simulink model "Group7_rotate"  (R2022a)
settings: Solver=FixedStepDiscrete  StartTime=0.0  StopTime=10  FixedStep=0.01  RelTol=1e-3
values from neighbouring files (symbols this model uses):
  axleLength = 0.136    [robotParameters.m]
  ticksPerRot = 20    [robotParameters.m]
  wheelR = 0.031    [robotParameters.m]
undefined symbols (not defined in the file or in its folder): DiscIntNeverNeededParam, InputPWM, lineLength, WheelSpeed
libraries: mobileRoboticsTrainingLib x4, slpidlib x1
settings Model: Creator=heath  LastModifiedBy=heath

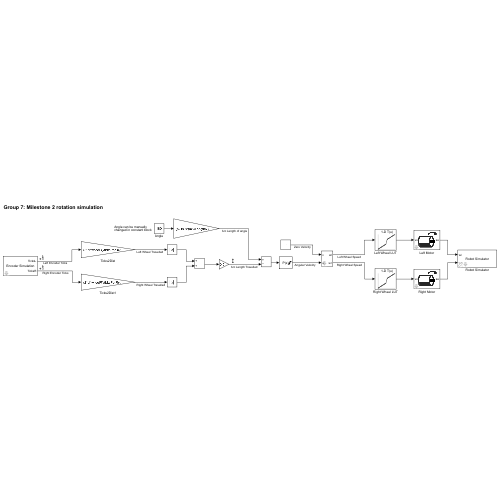
[thumbnail: Simulink's stored preview of the top-level diagram]
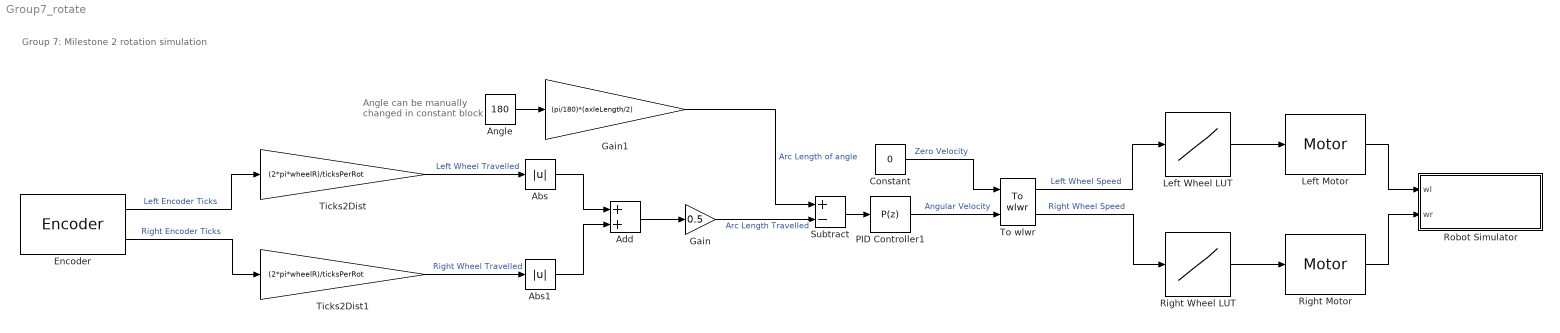
== system Group7_rotate ==
  note: Angle can be manually
      | changed in constant block
  note: Group 7: Milestone 2 rotation simulation
  Abs : Abs  SaturateOnIntegerOverflow=off
  Abs1 : Abs  SaturateOnIntegerOverflow=off
  Add : Sum
  Angle : Constant  Value=180
  Constant : Constant  Value=0
  Encoder : mobileRoboticsTrainingLib/Encoder  axleLength=axleLength  wheelR=wheelR  ticksPerRot=ticksPerRot
      settings: SourceProductName=Mobile Robotics Training Library
  Gain : Gain  Gain=0.5
  Gain1 : Gain  Gain=(pi/180)*(axleLength/2)
  Left Motor : mobileRoboticsTrainingLib/Motor  motorPlant=wheelMotorModel  sensorType=Speed
      settings: SourceProductName=Mobile Robotics Training Library
  Left Wheel LUT : Lookup_n-D  NumberOfTableDimensions=1  BreakpointsForDimension1=WheelSpeed  Table=InputPWM  InternalRulePriority=Speed  RndMeth=Simplest
  PID Controller1 : slpidlib/PID Controller  Controller=P  Form=Parallel  TimeDomain=Discrete-time  UseExternalTs=off  SampleTime=-1  IntegratorMethod=Forward Euler  FilterMethod=Forward Euler  ControllerParametersSource=internal  P=5  I=-4.46524084533701  UseKiTs=off  D=-0.502126631205415  N=20.6444730628157  UseFilter=on  TunerSelectOption=Transfer Function Based (PID Tuner App)  InitialConditionSource=internal  InitialConditionForIntegrator=0  InitialConditionForFilter=0  DifferentiatorICPrevScaledInput=0  ExternalReset=none  TrackingMode=off  Kt=1  LimitOutput=on  SatLimitsSource=internal  UpperSaturationLimit=16.67  LowerSaturationLimit=-16.67  LinearizeAsGain=on  AntiWindupMode=clamping  Kb=1  POutMin=[]  POutMax=[]  IOutMin=[]  IOutMax=[]  DOutMin=[]  DOutMax=[]  NOutMin=[]  NOutMax=[]  SumOutMin=[]  SumOutMax=[]  SaturationOutMin=[]  SaturationOutMax=[]  PParamMin=[]  PParamMax=[]  IParamMin=[]  IParamMax=[]  DParamMin=[]  DParamMax=[]  NParamMin=[]  NParamMax=[]  KbParamMin=[]  KbParamMax=[]  KtParamMin=[]  KtParamMax=[]  KbOutMin=[]  KbOutMax=[]  KtOutMin=[]  KtOutMax=[]  IntegratorOutMin=[]  IntegratorOutMax=[]  FilterOutMin=[]  FilterOutMax=[]  SumI1OutMin=[]  SumI1OutMax=[]  SumI2OutMin=[]  SumI2OutMax=[]  SumI3OutMin=[]  SumI3OutMax=[]  SumI4OutMin=[]  SumI4OutMax=[]  SumDOutMin=[]  SumDOutMax=[]  DifferentiatorOutMin=[]  DifferentiatorOutMax=[]  FilterDiffOutCoefMin=[]  FilterDiffOutCoefMax=[]  ReciprocalOutMin=[]  ReciprocalOutMax=[]  SumDenOutMin=[]  SumDenOutMax=[]  SumNumOutMin=[]  SumNumOutMax=[]  DivideOutMin=[]  DivideOutMax=[]  UdiffTsProdOutMin=[]  UdiffTsProdOutMax=[]  NTsProdOutMin=[]  NTsProdOutMax=[]  UintegralTsProdOutMin=[]  UintegralTsProdOutMax=[]  UngainTsProdOutMin=[]  UngainTsProdOutMax=[]  IntegratorContinuousStateAttributes=''  IntegratorStateMustResolveToSignalObject=off  IntegratorRTWStateStorageClass=Auto  FilterContinuousStateAttributes=''  FilterStateMustResolveToSignalObject=off  FilterRTWStateStorageClass=Auto  ParallelPVariant=InternalParameters  IdealPVariant=Disabled  IVariant=Disabled  DVariant=Disabled  IntegratorVariant=Disabled  SatVariant=Enabled  AWVariant=Disabled  PCopyVariant=Disabled  TRVariant=Disabled  FdbkBlocksVariant=Forward  IdealPFdbkVariant=Disabled  SatFdbkVariant=Disabled  DerivativeFilterVariant=Disabled  NVariant=Disabled  NCopyVariant=Disabled_SignalSpec  FilterICVariant=Disabled  IntegratorICVariant=Disabled  ExternalResetVariant=Disabled  TRSumVariant=Passthrough  SumFdbkVariant=Disabled  SumVariant=Passthrough_P  TsampFilterVariant=InternalTs  TsampNgainVariant=Passthrough  TsampIntegralVariant=Disabled_SignalSpec  ExternalSaturationOutDataTypeStr=Inherit: Same as second input  aMode=0
  Right Motor : mobileRoboticsTrainingLib/Motor  motorPlant=wheelMotorModel  sensorType=Speed
      settings: SourceProductName=Mobile Robotics Training Library
  Right Wheel LUT : Lookup_n-D  NumberOfTableDimensions=1  BreakpointsForDimension1=WheelSpeed  Table=InputPWM  InternalRulePriority=Speed  RndMeth=Simplest
  Robot Simulator : Subsystem  Priority=99  AncestorBlock=mobileRoboticsTrainingLib/Robot Simulator  mask(Robot Simulator){mapVar=[], startX=1, startY=1, startTheta=0, axleLength=axleLength, wheelR=wheelR}
      mask prompts: mapVar "Map Variable"; startX "Start X (m)"; startY "Start Y (m)"; startTheta "Theta (deg)"; axleLength "Axle Length (m)"; wheelR "Wheel Radius (m)"
      mask help: Configure robot simulator to use custom simulation maps and simulate closed-loop mobile robotics systems along with appropriate sensor simulation blocks.
      mask init:
      | set_param(bdroot,'SolverType','Fixed-Step');
      | set_param(bdroot,'Solver','FixedStepDiscrete');
      | 
      | if (exist('Ts'))
      |     set_param(bdroot,'FixedStep','Ts');
      | else
      |     set_param(bdroot,'FixedStep','0.01');
      | end
      | 
      | h = findobj('Name','Robot Simulator');
      | if ~isempty(h)
      |     close (h);
      | end
      | setupRobotSim();
      mask Help: web('Robot Simulator.htm')
      mask DialogControl mapCont Prompt: Map Setup
      mask DialogControl initPosCont Prompt: Initial Position
      mask DialogControl setPos Prompt: Set position interactively
      mask DialogControl setPos Callback:
      | %% Set starting point
      | setStartingPoint();
      mask DialogControl initOrientation Prompt: Initial Orientation
      mask DialogControl robotCharCont Prompt: Robot Characteristics
      mask Display: disp('Robot Simulator')
  Subtract : Sum  Inputs=+-
  Ticks2Dist : Gain  Gain=(2*pi*wheelR)/ticksPerRot
  Ticks2Dist1 : Gain  Gain=(2*pi*wheelR)/ticksPerRot
  To wlwr : mobileRoboticsTrainingLib/To wlwr  axleLength=axleLength  wheelR=wheelR
  wires:
  Ticks2Dist/1 -> Abs/1  "Left Wheel Travelled"
  Encoder/1 -> Ticks2Dist/1  "Left Encoder Ticks"
  Encoder/2 -> Ticks2Dist1/1  "Right Encoder Ticks"
  Ticks2Dist1/1 -> Abs1/1  "Right Wheel Travelled"
  Add/1 -> Gain/1
  Gain/1 -> Subtract/2  "Arc Length Travelled"
  PID Controller1/1 -> To wlwr/2  "Angular Velocity"
  To wlwr/1 -> Left Wheel LUT/1  "Left Wheel Speed"
  Left Wheel LUT/1 -> Left Motor/1
  To wlwr/2 -> Right Wheel LUT/1  "Right Wheel Speed"
  Right Wheel LUT/1 -> Right Motor/1
  Right Motor/1 -> Robot Simulator/2(wr)
  Left Motor/1 -> Robot Simulator/1(wl)
  Angle/1 -> Gain1/1
  Subtract/1 -> PID Controller1/1
  Abs/1 -> Add/1
  Abs1/1 -> Add/2
  Constant/1 -> To wlwr/1  "Zero Velocity"
  Gain1/1 -> Subtract/1  "Arc Length of angle"

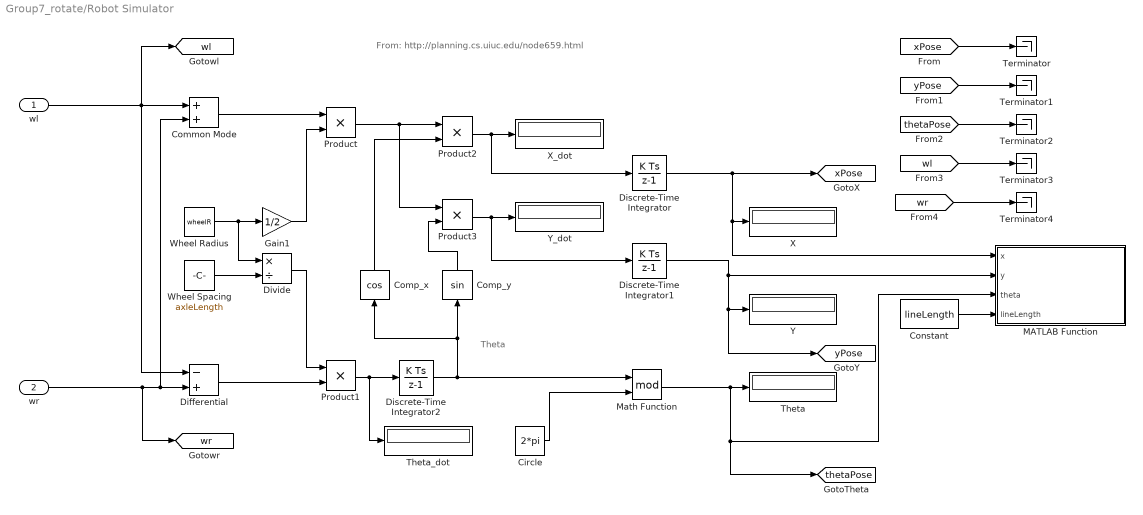
== system Group7_rotate/Robot Simulator ==
  note: Theta
  note: From: http://planning.cs.uiuc.edu/node659.html
  wl : Inport
  wr : Inport  Port=2
  Circle : Constant  Value=2*pi
  Common Mode : Sum
  Comp_x : Trigonometry  Operator=cos
  Comp_y : Trigonometry
  Constant : Constant  Value=lineLength
  Differential : Sum  Inputs=-+
  Discrete-Time Integrator : DiscreteIntegrator  InitialCondition=startX  SampleTime=-1  ICPrevOutput=DiscIntNeverNeededParam  ICPrevScaledInput=DiscIntNeverNeededParam
  Discrete-Time Integrator1 : DiscreteIntegrator  InitialCondition=startY  SampleTime=-1  ICPrevOutput=DiscIntNeverNeededParam  ICPrevScaledInput=DiscIntNeverNeededParam
  Discrete-Time Integrator2 : DiscreteIntegrator  InitialCondition=startTheta*(pi/180)  SampleTime=-1  ICPrevOutput=DiscIntNeverNeededParam  ICPrevScaledInput=DiscIntNeverNeededParam
  Divide : Product  Inputs=*/
  Gain1 : Gain  Gain=1/2
  MATLAB Function : MATLAB Function  TreatAsAtomicUnit=on
  Math Function : Math  Operator=mod  SignedPower=on
  Product{,1..3} (4 alike) : Product  RndMeth=Zero
  Terminator{,1..4} (5 alike) : Terminator
  Theta : Display
  Theta_dot : Display
  Wheel Radius : Constant  Value=wheelR
  Wheel Spacing : Constant  Value=axleLength
  X : Display
  X_dot : Display
  Y : Display
  Y_dot : Display
  tag scope: thetaPose=global, wl=global, wr=global, xPose=global, yPose=global
  wires:
  [wr] -> Terminator4/1
  [wl] -> Terminator3/1
  Math Function/1 -> [thetaPose], MATLAB Function/3(theta), Theta/1
  Differential/1 -> Product1/2
  Comp_y/1 -> Product3/2
  Discrete-Time Integrator/1 -> [xPose], MATLAB Function/1(x), X/1
  Product3/1 -> Discrete-Time Integrator1/1, Y_dot/1
  Discrete-Time Integrator1/1 -> Y/1, [yPose], MATLAB Function/2(y)
  Divide/1 -> Product1/1
  wr/1 -> [wr], Common Mode/2, Differential/2
  Discrete-Time Integrator2/1 -> Math Function/1, Comp_x/1, Comp_y/1
  wl/1 -> [wl], Common Mode/1, Differential/1
  Comp_x/1 -> Product2/2
  Product1/1 -> Discrete-Time Integrator2/1, Theta_dot/1
  Wheel Radius/1 -> Divide/1, Gain1/1
  Wheel Spacing/1 -> Divide/2
  Product2/1 -> Discrete-Time Integrator/1, X_dot/1
  Gain1/1 -> Product/2
  Common Mode/1 -> Product/1
  Product/1 -> Product3/1, Product2/1
  Circle/1 -> Math Function/2
  Constant/1 -> MATLAB Function/4(lineLength)
  [xPose] -> Terminator/1
  [yPose] -> Terminator1/1
  [thetaPose] -> Terminator2/1

== matlab function Group7_rotate/Robot Simulator/MATLAB Function ==
  data: x input; y input; theta input; lineLength input
function plotRobot(x,y,theta,lineLength)
% Get plot details
coder.extrinsic('evalin','plot')
ph1 = evalin('base','PlotHandle1');
ph2 = evalin('base','PlotHandle2');

% Find length orientation line
xp = [x x+lineLength*cos(theta)];
yp = [y y+lineLength*sin(theta)];

% Plot robot
set(ph1,'xdata',xp,'ydata',yp);
set(ph2,'xdata',x,'ydata',y);
drawnow('limitrate')
